simulink model "quanser_heli_IdentificadorRHONN"  (R2025a)
settings: Solver=FixedStepAuto  StartTime=0.0  StopTime=15  FixedStep=.001  RelTol=1e-3
values from neighbouring files (symbols this model uses):
  P1 = eye(2)*5e2    [ParametrosRHONN.m]
  P12 = eye(4)*5e2    [ParametrosRHONN.m]
  P2 = eye(2)*5e2    [ParametrosRHONN.m]
  P22 = eye(4)*5e2    [ParametrosRHONN.m]
  P3 = eye(2)*5e2    [ParametrosRHONN.m]
  P32 = eye(4)*5e2    [ParametrosRHONN.m]
  P4 = eye(2)*5e2    [ParametrosRHONN.m]
  P42 = eye(4)*5e2    [ParametrosRHONN.m]
  theta_0 = -40.5*pi/180    (= -0.706858347058)    [setup_heli_2d_base.m]
  VMAX_UPM_P = 24    [setup_heli_2d_base.m]
  VMAX_UPM_Y = 15    [setup_heli_2d_base.m]
  wk = zeros(8,1)    [ParametrosRHONN.m]
  wk2 = zeros(16,1)    [ParametrosRHONN.m]
undefined symbols (not defined in the file or in its folder): B_p, B_y, dspblkCoreblockFVToolHelper, g, gcbh, J_eq_p, J_eq_y, K_pp, K_py, K_yp, K_yy, l_cm, m_heli
libraries: simulink x2
settings Model: Creator=aceve  LastModifiedBy=aceve

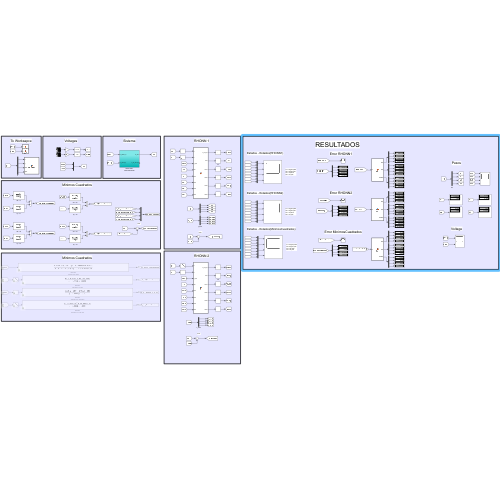
[thumbnail: Simulink's stored preview of the top-level diagram]
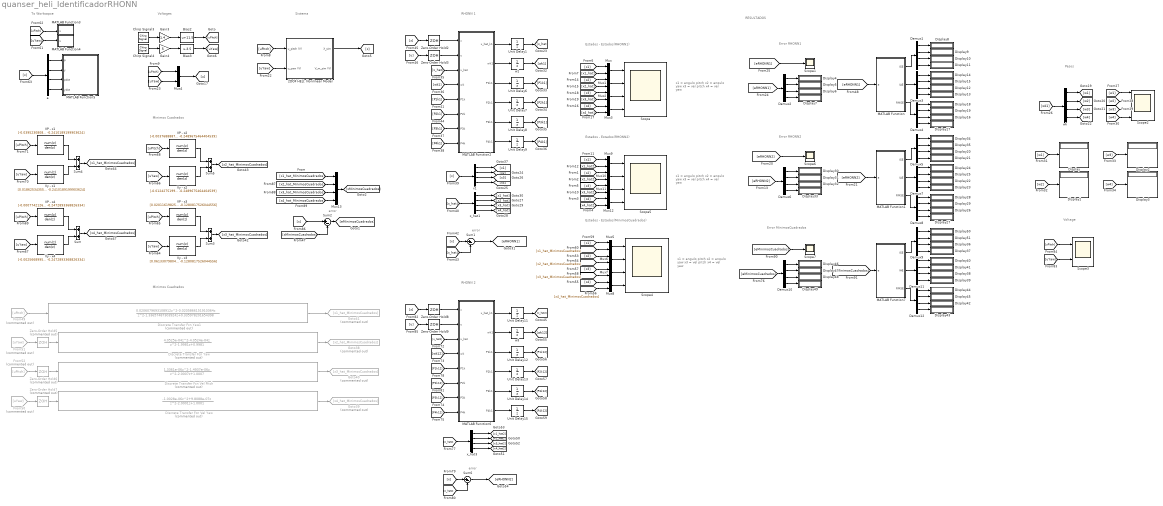
== system quanser_heli_IdentificadorRHONN ==
  note: Estados - Estados(RHONN1)
  note: Error RHONN1
  note: x1 = angulo pitch
      | x2 = angulo yaw
      | x3 = vel pitch
      | x4 = vel yaw
  note: Voltages
  note: Sistema
  note: RESULTADOS
  note: Pesos
  note: error
  note: RHONN 1
  note: Voltage
  note: Minimos Cuadrados
  note: Estados - Estados(MinimosCuadrados)
  note: x1 = angulo pitch
      | x2 = angulo yaw
      | x3 = vel pitch
      | x4 = vel yaw
  note: To Worksapce
  note: Minimos Cuadrados
  note: error
  note: RHONN 2
  note: Estados - Estados(RHONN2)
  note: x1 = angulo pitch
      | x2 = angulo yaw
      | x3 = vel pitch
      | x4 = vel yaw
  note: Error RHONN2
  note: error
  note: Error MinimosCuadrados
  2DOF HELI: Nonlinear Model : Subsystem
  Bias2 : Bias  Bias=11.5  SaturateOnIntegerOverflow=off
  Bias3 : Bias  Bias=-3.5  SaturateOnIntegerOverflow=off
  Chirp Signal3 : simulink/Sources/Chirp Signal  f1=0.08  T=10  f2=1
  Chirp Signal4 : simulink/Sources/Chirp Signal  f1=0.05  T=100  f2=1
  Demux{1..12} (12 alike) : Demux
  Discrete Transfer Fcn Vel Pitch : DiscreteTransferFcn  Commented=on  LoadFcn=dspblkCoreblockFVToolHelper(gcbh,'load');  Numerator=[1.3361e-06 -1.4937e-06 0]  Denominator=[1 -2.0007 1.0007]  a0EqualsOne=on
      settings: CopyFcn=dspblkCoreblockFVToolHelper(gcbh,'copy');  DeleteFcn=dspblkCoreblockFVToolHelper(gcbh,'close');  ModelCloseFcn=dspblkCoreblockFVToolHelper(gcbh,'close');  PreSaveFcn=dspblkCoreblockFVToolHelper(gcbh,'presave');  PostSaveFcn=dspblkCoreblockFVToolHelper(gcbh,'postsave');  CloseFcn=dspblkCoreblockFVToolHelper(gcbh,'close');
  Discrete Transfer Fcn Vel Yaw : DiscreteTransferFcn  Commented=on  LoadFcn=dspblkCoreblockFVToolHelper(gcbh,'load');  Numerator=[-1.0028e-06 9.8088e-07 0]  Denominator=[1 -2.0001 1.0001]  a0EqualsOne=on
      settings: CopyFcn=dspblkCoreblockFVToolHelper(gcbh,'copy');  DeleteFcn=dspblkCoreblockFVToolHelper(gcbh,'close');  ModelCloseFcn=dspblkCoreblockFVToolHelper(gcbh,'close');  PreSaveFcn=dspblkCoreblockFVToolHelper(gcbh,'presave');  PostSaveFcn=dspblkCoreblockFVToolHelper(gcbh,'postsave');  CloseFcn=dspblkCoreblockFVToolHelper(gcbh,'close');
  Discrete Transfer Fcn Yaw : DiscreteTransferFcn  Commented=on  LoadFcn=dspblkCoreblockFVToolHelper(gcbh,'load');  Numerator=[4.0525e-04 -4.0524e-04 0]  Denominator=[1 -1.9981 0.9981]  a0EqualsOne=on
      settings: CopyFcn=dspblkCoreblockFVToolHelper(gcbh,'copy');  DeleteFcn=dspblkCoreblockFVToolHelper(gcbh,'close');  ModelCloseFcn=dspblkCoreblockFVToolHelper(gcbh,'close');  PreSaveFcn=dspblkCoreblockFVToolHelper(gcbh,'presave');  PostSaveFcn=dspblkCoreblockFVToolHelper(gcbh,'postsave');  CloseFcn=dspblkCoreblockFVToolHelper(gcbh,'close');
  Discrete Transfer Fcn Yaw1 : DiscreteTransferFcn  Commented=on  LoadFcn=dspblkCoreblockFVToolHelper(gcbh,'load');  Numerator=[0.0206079693108912 -0.0205866151910364 0]  Denominator=[1 -1.33657487303924 0.335978201654398]  InitialStates=[-0.61509767 0.12995987]  a0EqualsOne=on
      settings: CopyFcn=dspblkCoreblockFVToolHelper(gcbh,'copy');  DeleteFcn=dspblkCoreblockFVToolHelper(gcbh,'close');  ModelCloseFcn=dspblkCoreblockFVToolHelper(gcbh,'close');  PreSaveFcn=dspblkCoreblockFVToolHelper(gcbh,'presave');  PostSaveFcn=dspblkCoreblockFVToolHelper(gcbh,'postsave');  CloseFcn=dspblkCoreblockFVToolHelper(gcbh,'close');
  Display{,1..51} (52 alike) : Display
  From49 : From  Commented=on  GotoTag=uPitch
  From50 : From  Commented=on  GotoTag=uYaw
  From51 : From  Commented=on  GotoTag=uYaw
  From52 : From  Commented=on  GotoTag=uPitch
  Gain3 : Gain  Gain=1.4
  Gain4 : Gain  Gain=5
  Goto38 : Goto  Commented=on  GotoTag=x2_hat_MinimosCuadrados
  Goto39 : Goto  Commented=on  GotoTag=x4_hat_MinimosCuadrados
  Goto40 : Goto  Commented=on  GotoTag=x3_hat_MinimosCuadrados
  Goto41 : Goto  Commented=on  GotoTag=x1_hat_MinimosCuadrados
  MATLAB Function : MATLAB Function  TreatAsAtomicUnit=on
  MATLAB Function1 : MATLAB Function  TreatAsAtomicUnit=on
  MATLAB Function2 : MATLAB Function  TreatAsAtomicUnit=on
  MATLAB Function3 : MATLAB Function  TreatAsAtomicUnit=on
  MATLAB Function4 : MATLAB Function  TreatAsAtomicUnit=on
  MATLAB Function5 : MATLAB Function  TreatAsAtomicUnit=on
  MATLAB Function6 : MATLAB Function  TreatAsAtomicUnit=on
  MATLAB Function7 : MATLAB Function  TreatAsAtomicUnit=on
  Mux{,1..12} (13 alike) : Mux  Inputs=2
  Mux13 : Mux
  Scope{,2,4..5} (4 alike) : Scope  NumInputPorts=4
      Scope settings: ActiveDisplayYMinimum=-0.84384917353702449  ActiveDisplayYMaximum=0.094948446572447137
      Scope2 settings: ActiveDisplayYMinimum=-0.70088433050936716  ActiveDisplayYMaximum=1.4334945118996132  DataLoggingVariableName=ScopeData2
      Scope4 settings: ActiveDisplayYMinimum=-0.77876884866635865  ActiveDisplayYMaximum=-0.059663832579807244  DataLoggingVariableName=ScopeData4
      Scope5 settings: ActiveDisplayYMinimum=-0.84384917353702449  ActiveDisplayYMaximum=0.094948446572447137  DataLoggingVariableName=ScopeData5
  Scope1 : Scope
      settings: ActiveDisplayYMinimum=-0.80920578422516953  ActiveDisplayYMaximum=0.12318319700603184
  Scope3 : Scope  NumInputPorts=2
      settings: ActiveDisplayYMinimum=-11.174999961452089  ActiveDisplayYMaximum=15.574999929221228  DataLoggingVariableName=ScopeData3
  Scope6 : Scope
      settings: ActiveDisplayYMinimum=-0.80920578422516953  ActiveDisplayYMaximum=0.12318319700603184  DataLoggingVariableName=ScopeData6
  Scope7 : Scope
      settings: ActiveDisplayYMinimum=-0.80920578422516953  ActiveDisplayYMaximum=0.12318319700603184  DataLoggingVariableName=ScopeData7
  Sum{,3..5} (4 alike) : Sum
  Sum1 : Sum  Inputs=|+-
  Sum2 : Sum  Inputs=|+-
  Sum6 : Sum  Inputs=|+-
  Unit Delay1 : UnitDelay  SampleTime=-1  HasFrameUpgradeWarning=on
  Unit Delay11 : UnitDelay  SampleTime=-1  HasFrameUpgradeWarning=on
  Unit Delay12 : UnitDelay  InitialCondition=P12  SampleTime=-1  HasFrameUpgradeWarning=on
  Unit Delay13 : UnitDelay  InitialCondition=P22  SampleTime=-1  HasFrameUpgradeWarning=on
  Unit Delay14 : UnitDelay  InitialCondition=P32  SampleTime=-1  HasFrameUpgradeWarning=on
  Unit Delay15 : UnitDelay  InitialCondition=P42  SampleTime=-1  HasFrameUpgradeWarning=on
  Unit Delay6 : UnitDelay  InitialCondition=P1  SampleTime=-1  HasFrameUpgradeWarning=on
  Unit Delay7 : UnitDelay  InitialCondition=P2  SampleTime=-1  HasFrameUpgradeWarning=on
  Unit Delay8 : UnitDelay  InitialCondition=P3  SampleTime=-1  HasFrameUpgradeWarning=on
  Unit Delay9 : UnitDelay  InitialCondition=P4  SampleTime=-1  HasFrameUpgradeWarning=on
  VP - x1 : DiscreteTransferFcn  LoadFcn=dspblkCoreblockFVToolHelper(gcbh,'load');  Numerator=[-0.03952308083807093 0.01457910362503944 0.0132465358893853 0.0116502395543983 0]  Denominator=[1 -0.2596941129912199 -0.2512083520588688 -0.246113610865054 -0.2410189199903624]  a0EqualsOne=on
      settings: CopyFcn=dspblkCoreblockFVToolHelper(gcbh,'copy');  DeleteFcn=dspblkCoreblockFVToolHelper(gcbh,'close');  ModelCloseFcn=dspblkCoreblockFVToolHelper(gcbh,'close');  PreSaveFcn=dspblkCoreblockFVToolHelper(gcbh,'presave');  PostSaveFcn=dspblkCoreblockFVToolHelper(gcbh,'postsave');  CloseFcn=dspblkCoreblockFVToolHelper(gcbh,'close');
  VP - x2 : DiscreteTransferFcn  LoadFcn=dspblkCoreblockFVToolHelper(gcbh,'load');  Numerator=[-0.003768888777310456 -0.001235966092478362 0.001315157335725626 0.003827291194365801 0]  Denominator=[1 -0.2509050215084465 -0.2502617960478971 -0.2496159714324903 -0.2489675464404539]  a0EqualsOne=on
      settings: CopyFcn=dspblkCoreblockFVToolHelper(gcbh,'copy');  DeleteFcn=dspblkCoreblockFVToolHelper(gcbh,'close');  ModelCloseFcn=dspblkCoreblockFVToolHelper(gcbh,'close');  PreSaveFcn=dspblkCoreblockFVToolHelper(gcbh,'presave');  PostSaveFcn=dspblkCoreblockFVToolHelper(gcbh,'postsave');  CloseFcn=dspblkCoreblockFVToolHelper(gcbh,'close');
  VP - x3 : DiscreteTransferFcn  LoadFcn=dspblkCoreblockFVToolHelper(gcbh,'load');  Numerator=[0.02011619825005108 0.006568459415468767 -0.006119667445303119 -0.02055837664883229 0]  Denominator=[1 -0.3716516698733148 -0.2906441537001457 -0.2094533609274164 -0.1280817526044556]  a0EqualsOne=on
      settings: CopyFcn=dspblkCoreblockFVToolHelper(gcbh,'copy');  DeleteFcn=dspblkCoreblockFVToolHelper(gcbh,'close');  ModelCloseFcn=dspblkCoreblockFVToolHelper(gcbh,'close');  PreSaveFcn=dspblkCoreblockFVToolHelper(gcbh,'presave');  PostSaveFcn=dspblkCoreblockFVToolHelper(gcbh,'postsave');  CloseFcn=dspblkCoreblockFVToolHelper(gcbh,'close');
  VP - x4 : DiscreteTransferFcn  LoadFcn=dspblkCoreblockFVToolHelper(gcbh,'load');  Numerator=[-0.000774212667988009 -0.0001464440180138851 0.0004853777300417859 0.001107287718628923 0]  Denominator=[1 -0.2478215083584044 -0.2476467681554213 -0.2474693715809018 -0.2472893368826334]  a0EqualsOne=on
      settings: CopyFcn=dspblkCoreblockFVToolHelper(gcbh,'copy');  DeleteFcn=dspblkCoreblockFVToolHelper(gcbh,'close');  ModelCloseFcn=dspblkCoreblockFVToolHelper(gcbh,'close');  PreSaveFcn=dspblkCoreblockFVToolHelper(gcbh,'presave');  PostSaveFcn=dspblkCoreblockFVToolHelper(gcbh,'postsave');  CloseFcn=dspblkCoreblockFVToolHelper(gcbh,'close');
  Vy - x1 : DiscreteTransferFcn  LoadFcn=dspblkCoreblockFVToolHelper(gcbh,'load');  Numerator=[0.01862534355611094 -0.002149223852187077 -0.006182902374224723 -0.01026641731777086 0]  Denominator=[1 -0.2596941129912199 -0.2512083520588688 -0.246113610865054 -0.2410189199903624]  a0EqualsOne=on
      settings: CopyFcn=dspblkCoreblockFVToolHelper(gcbh,'copy');  DeleteFcn=dspblkCoreblockFVToolHelper(gcbh,'close');  ModelCloseFcn=dspblkCoreblockFVToolHelper(gcbh,'close');  PreSaveFcn=dspblkCoreblockFVToolHelper(gcbh,'presave');  PostSaveFcn=dspblkCoreblockFVToolHelper(gcbh,'postsave');  CloseFcn=dspblkCoreblockFVToolHelper(gcbh,'close');
  Vy - x2 : DiscreteTransferFcn  LoadFcn=dspblkCoreblockFVToolHelper(gcbh,'load');  Numerator=[-0.0124275199058459 -0.004066593005302975 0.00431430457234765 0.01273262520586928 0]  Denominator=[1 -0.2509050215084465 -0.2502617960478971 -0.2496159714324903 -0.2489675464404539]  a0EqualsOne=on
      settings: CopyFcn=dspblkCoreblockFVToolHelper(gcbh,'copy');  DeleteFcn=dspblkCoreblockFVToolHelper(gcbh,'close');  ModelCloseFcn=dspblkCoreblockFVToolHelper(gcbh,'close');  PreSaveFcn=dspblkCoreblockFVToolHelper(gcbh,'presave');  PostSaveFcn=dspblkCoreblockFVToolHelper(gcbh,'postsave');  CloseFcn=dspblkCoreblockFVToolHelper(gcbh,'close');
  Vy - x3 : DiscreteTransferFcn  LoadFcn=dspblkCoreblockFVToolHelper(gcbh,'load');  Numerator=[0.06133079804282214 0.0207651122165453 -0.02048820045618499 -0.06163048150396479 0]  Denominator=[1 -0.3716516698733148 -0.2906441537001457 -0.2094533609274164 -0.1280817526044556]  a0EqualsOne=on
      settings: CopyFcn=dspblkCoreblockFVToolHelper(gcbh,'copy');  DeleteFcn=dspblkCoreblockFVToolHelper(gcbh,'close');  ModelCloseFcn=dspblkCoreblockFVToolHelper(gcbh,'close');  PreSaveFcn=dspblkCoreblockFVToolHelper(gcbh,'presave');  PostSaveFcn=dspblkCoreblockFVToolHelper(gcbh,'postsave');  CloseFcn=dspblkCoreblockFVToolHelper(gcbh,'close');
  Vy - x4 : DiscreteTransferFcn  LoadFcn=dspblkCoreblockFVToolHelper(gcbh,'load');  Numerator=[-0.002566899592150418 -0.0004840187454093538 0.001591783821110975 0.003664753148714413 0]  Denominator=[1 -0.2478215083584044 -0.2476467681554213 -0.2474693715809018 -0.2472893368826334]  a0EqualsOne=on
      settings: CopyFcn=dspblkCoreblockFVToolHelper(gcbh,'copy');  DeleteFcn=dspblkCoreblockFVToolHelper(gcbh,'close');  ModelCloseFcn=dspblkCoreblockFVToolHelper(gcbh,'close');  PreSaveFcn=dspblkCoreblockFVToolHelper(gcbh,'presave');  PostSaveFcn=dspblkCoreblockFVToolHelper(gcbh,'postsave');  CloseFcn=dspblkCoreblockFVToolHelper(gcbh,'close');
  Zero-Order Hold{2..3,8..9} (4 alike) : ZeroOrderHold  SampleTime=-1
  Zero-Order Hold5 : ZeroOrderHold  Commented=on  SampleTime=-1
  Zero-Order Hold6 : ZeroOrderHold  Commented=on  SampleTime=-1
  Zero-Order Hold7 : ZeroOrderHold  Commented=on  SampleTime=-1
  a : Demux
  w1 : UnitDelay  InitialCondition=[wk]  SampleTime=-1  HasFrameUpgradeWarning=on
  w3 : UnitDelay  InitialCondition=[wk2]  SampleTime=-1  HasFrameUpgradeWarning=on
  wk : Demux
  x1 : Demux
  x_hat1 : Demux
  x_hat3 : Demux
  wires:
  2DOF HELI: Nonlinear Model/1(X_sim) -> [x]
  Mux/1 -> Scope/1
  Mux1/1 -> Scope/2
  Mux2/1 -> Scope/3
  Mux3/1 -> Scope/4
  [x1] -> Mux/1
  [x1_hat] -> Mux/2
  [x2] -> Mux1/1
  [x2_hat] -> Mux1/2
  [x4] -> Mux3/1
  [x4_hat] -> Mux3/2
  [x3] -> Mux2/1
  [x3_hat] -> Mux2/2
  Chirp Signal3/1 -> Gain3/1
  Gain3/1 -> Bias2/1
  Chirp Signal4/1 -> Gain4/1
  Gain4/1 -> Bias3/1
  Bias2/1 -> [uPitch]
  Bias3/1 -> [uYaw]
  [uPitch] -> 2DOF HELI: Nonlinear Model/1(u_pitch (V))
  [uYaw] -> 2DOF HELI: Nonlinear Model/2(u_yaw (V))
  [uPitch] -> Mux4/1
  [uYaw] -> Mux4/2
  [eRHONN1] -> Demux2/1
  Demux2/2 -> Display5/1
  Demux2/4 -> Display7/1
  Demux2/1 -> Display4/1
  Demux2/3 -> Display6/1
  [eRHONN1] -> Scope1/1
  [wk1] -> wk/1
  wk/1 -> [w1]
  wk/2 -> [w2]
  wk/4 -> [w4]
  wk/3 -> [w3]
  [w1] -> Scope2/1
  [w2] -> Scope2/2
  [w4] -> Scope2/4
  [w3] -> Scope2/3
  [w1] -> Display/1
  [w2] -> Display1/1
  [w3] -> Display2/1
  [w4] -> Display3/1
  [x_hat] -> x_hat1/1
  MATLAB Function2/5(P3k1) -> Unit Delay8/1
  Unit Delay1/1 -> [x_hat]
  x1/2 -> [x2]
  x_hat1/3 -> [x3_hat]
  MATLAB Function2/2(wk1) -> w1/1
  [x] -> Zero-Order Hold2/1
  [x_hat] -> MATLAB Function2/3(x_hat)
  [P3k1] -> MATLAB Function2/7(P3k)
  [u] -> Zero-Order Hold3/1
  MATLAB Function2/1(x_hat_k1) -> Unit Delay1/1
  x1/4 -> [x4]
  [P2k1] -> MATLAB Function2/6(P2k)
  MATLAB Function2/6(P4k1) -> Unit Delay9/1
  x_hat1/1 -> [x1_hat]
  MATLAB Function2/4(P2k1) -> Unit Delay7/1
  Zero-Order Hold3/1 -> MATLAB Function2/2(u)
  x_hat1/4 -> [x4_hat]
  Zero-Order Hold2/1 -> MATLAB Function2/1(x)
  [x_hat] -> Sum1/2
  Unit Delay9/1 -> [P4k1]
  [wk1] -> MATLAB Function2/4(wk)
  w1/1 -> [wk1]
  [x] -> x1/1
  x1/1 -> [x1]
  x1/3 -> [x3]
  [P4k1] -> MATLAB Function2/8(P4k)
  [P1k1] -> MATLAB Function2/5(P1k)
  Sum1/1 -> [eRHONN1]
  Unit Delay7/1 -> [P2k1]
  Unit Delay8/1 -> [P3k1]
  Unit Delay6/1 -> [P1k1]
  MATLAB Function2/3(P1k1) -> Unit Delay6/1
  x_hat1/2 -> [x2_hat]
  [x] -> Sum1/1
  [uYaw] -> Scope3/2
  [uPitch] -> Scope3/1
  Mux4/1 -> [u]
  [eRHONN1] -> MATLAB Function/1(e)
  Demux1/4 -> Display11/1
  Demux1/3 -> Display10/1
  Demux1/2 -> Display9/1
  Demux1/1 -> Display8/1
  Demux3/4 -> Display13/1
  Demux3/2 -> Display15/1
  Demux3/3 -> Display12/1
  Demux3/1 -> Display14/1
  Demux4/3 -> Display16/1
  Demux4/4 -> Display17/1
  Demux4/2 -> Display19/1
  MATLAB Function/1(ISE) -> Demux1/1
  MATLAB Function/2(IAE) -> Demux3/1
  MATLAB Function/3(RMSE) -> Demux4/1
  Demux4/1 -> Display18/1
  Discrete Transfer Fcn Vel Yaw/1 -> Goto39/1
  Discrete Transfer Fcn Vel Pitch/1 -> Goto40/1
  Discrete Transfer Fcn Yaw/1 -> Goto38/1
  Mux8/1 -> Scope4/4
  [x3_hat_MinimosCuadrados] -> Mux7/2
  [x2_hat_MinimosCuadrados] -> Mux6/2
  [x3] -> Mux7/1
  Mux5/1 -> Scope4/1
  Mux7/1 -> Scope4/3
  [x2] -> Mux6/1
  [x4] -> Mux8/1
  Mux6/1 -> Scope4/2
  [x4_hat_MinimosCuadrados] -> Mux8/2
  [x1_hat_MinimosCuadrados] -> Mux5/2
  Zero-Order Hold5/1 -> Discrete Transfer Fcn Yaw/1
  Zero-Order Hold6/1 -> Discrete Transfer Fcn Vel Pitch/1
  Zero-Order Hold7/1 -> Discrete Transfer Fcn Vel Yaw/1
  [x1] -> Mux5/1
  [uPitch] -> MATLAB Function3/1(u)
  [uYaw] -> MATLAB Function4/1(u)
  [x] -> a/1
  a/1 -> MATLAB Function5/1(p)
  a/2 -> MATLAB Function5/2(y)
  a/3 -> MATLAB Function5/3(pdot)
  a/4 -> MATLAB Function5/4(ydot)
  From51/1 -> Zero-Order Hold5/1
  From50/1 -> Zero-Order Hold7/1
  From52/1 -> Zero-Order Hold6/1
  Discrete Transfer Fcn Yaw1/1 -> Goto41/1
  From49/1 -> Discrete Transfer Fcn Yaw1/1
  [uYaw] -> Vy - x4/1
  [uPitch] -> VP - x4/1
  Sum/1 -> [x4_hat_MinimosCuadrados]
  VP - x4/1 -> Sum/1
  Vy - x4/1 -> Sum/2
  [uPitch] -> VP - x3/1
  Sum3/1 -> [x3_hat_MinimosCuadrados]
  VP - x3/1 -> Sum3/1
  Vy - x3/1 -> Sum3/2
  [uYaw] -> Vy - x3/1
  [uPitch] -> VP - x1/1
  Sum4/1 -> [x1_hat_MinimosCuadrados]
  VP - x1/1 -> Sum4/1
  Vy - x1/1 -> Sum4/2
  VP - x2/1 -> Sum5/1
  [uPitch] -> VP - x2/1
  Sum5/1 -> [x2_hat_MinimosCuadrados]
  Vy - x2/1 -> Sum5/2
  [uYaw] -> Vy - x2/1
  [uYaw] -> Vy - x1/1
  w3/1 -> [wk12]
  Unit Delay13/1 -> [P2k12]
  MATLAB Function6/6(P4k1) -> Unit Delay15/1
  [x_hat2] -> Sum6/2
  Sum6/1 -> [eRHONN2]
  Unit Delay12/1 -> [P1k12]
  [u] -> Zero-Order Hold9/1
  Unit Delay11/1 -> [x_hat2]
  MATLAB Function6/4(P2k1) -> Unit Delay13/1
  x_hat3/1 -> [x1_hat2]
  Zero-Order Hold9/1 -> MATLAB Function6/2(u)
  [x] -> Sum6/1
  x_hat3/3 -> [x3_hat2]
  [x_hat2] -> x_hat3/1
  x_hat3/2 -> [x2_hat2]
  MATLAB Function6/2(wk1) -> w3/1
  [P4k12] -> MATLAB Function6/8(P4k)
  Unit Delay14/1 -> [P3k12]
  x_hat3/4 -> [x4_hat2]
  [wk12] -> MATLAB Function6/4(wk)
  [P3k12] -> MATLAB Function6/7(P3k)
  Zero-Order Hold8/1 -> MATLAB Function6/1(x)
  Unit Delay15/1 -> [P4k12]
  [P2k12] -> MATLAB Function6/6(P2k)
  [x_hat2] -> MATLAB Function6/3(x_hat)
  [P1k12] -> MATLAB Function6/5(P1k)
  MATLAB Function6/1(x_hat_k1) -> Unit Delay11/1
  MATLAB Function6/3(P1k1) -> Unit Delay12/1
  MATLAB Function6/5(P3k1) -> Unit Delay14/1
  [x] -> Zero-Order Hold8/1
  Mux11/1 -> Scope5/3
  [x2_hat2] -> Mux10/2
  Mux10/1 -> Scope5/2
  [x3] -> Mux11/1
  Mux9/1 -> Scope5/1
  [x2] -> Mux10/1
  [x4_hat2] -> Mux12/2
  [x3_hat2] -> Mux11/2
  [x4] -> Mux12/1
  [x1_hat2] -> Mux9/2
  Mux12/1 -> Scope5/4
  [x1] -> Mux9/1
  Demux5/3 -> Display20/1
  Demux6/1 -> Display30/1
  Demux5/4 -> Display21/1
  Demux7/1 -> Display24/1
  Demux5/2 -> Display35/1
  Demux8/1 -> Display28/1
  Demux8/3 -> Display26/1
  Demux6/4 -> Display33/1
  MATLAB Function1/2(IAE) -> Demux7/1
  Demux6/3 -> Display32/1
  Demux6/2 -> Display31/1
  MATLAB Function1/3(RMSE) -> Demux8/1
  Demux5/1 -> Display34/1
  Demux7/2 -> Display25/1
  [eRHONN2] -> Demux6/1
  [eRHONN2] -> MATLAB Function1/1(e)
  Demux8/4 -> Display27/1
  [eRHONN2] -> Scope6/1
  Demux7/4 -> Display23/1
  MATLAB Function1/1(ISE) -> Demux5/1
  Demux8/2 -> Display29/1
  Demux7/3 -> Display22/1
  Sum2/1 -> [eMinimosCuadrados]
  [x3_hat_MinimosCuadrados] -> Mux13/3
  [x2_hat_MinimosCuadrados] -> Mux13/2
  [x1_hat_MinimosCuadrados] -> Mux13/1
  [x4_hat_MinimosCuadrados] -> Mux13/4
  [x] -> Sum2/1
  [xMinimosCuadrados] -> Sum2/2
  [eMinimosCuadrados] -> MATLAB Function7/1(e)
  Demux11/3 -> Display38/1
  Demux12/2 -> Display45/1
  MATLAB Function7/1(ISE) -> Demux9/1
  Demux12/4 -> Display43/1
  Demux9/1 -> Display50/1
  [eMinimosCuadrados] -> Scope7/1
  [eMinimosCuadrados] -> Demux10/1
  Demux11/2 -> Display41/1
  Demux11/4 -> Display39/1
  Demux10/3 -> Display48/1
  Demux10/2 -> Display47/1
  MATLAB Function7/3(RMSE) -> Demux12/1
  Demux10/4 -> Display49/1
  Demux12/3 -> Display42/1
  Demux12/1 -> Display44/1
  Demux11/1 -> Display40/1
  Demux9/4 -> Display37/1
  Demux9/2 -> Display51/1
  Demux10/1 -> Display46/1
  MATLAB Function7/2(IAE) -> Demux11/1
  Demux9/3 -> Display36/1
  Mux13/1 -> [xMinimosCuadrados]

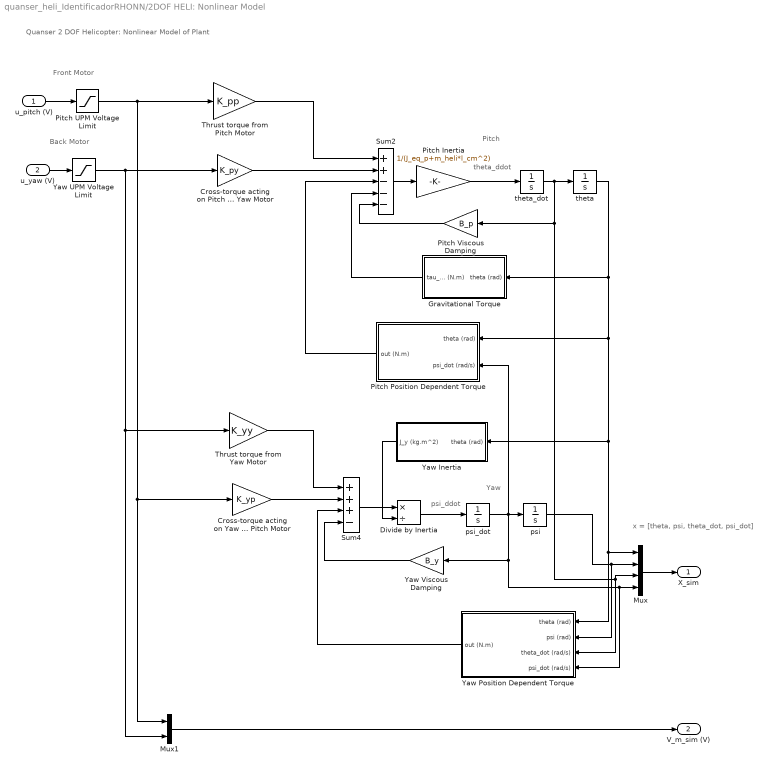
== system quanser_heli_IdentificadorRHONN/2DOF HELI: Nonlinear Model ==
  note: Back Motor
  note: Front Motor
  note: x = [theta, psi, theta_dot, psi_dot]
  note: Quanser 2 DOF Helicopter: Nonlinear Model of Plant
  note: theta_ddot
  note: psi_ddot
  note: Pitch
  note: Yaw
  u_pitch (V) : Inport
  u_yaw (V) : Inport  Port=2
  Cross-torque acting on Pitch from Yaw Motor : Gain  Gain=K_py
  Cross-torque acting on Yaw from Pitch Motor : Gain  Gain=K_yp
  Divide by Inertia : Product  Inputs=*/
  Gravitational Torque : Subsystem
  Mux : Mux
  Mux1 : Mux  Inputs=2
  Pitch Inertia : Gain  Gain=1/(J_eq_p+m_heli*l_cm^2)
  Pitch Position Dependent Torque : Subsystem  AncestorBlock=heli_2d_lib/2DOF Helicopter: Nonlinear Model/Yaw Nonlinear Element
  Pitch UPM Voltage Limit : Saturate  UpperLimit=VMAX_UPM_P  LowerLimit=- VMAX_UPM_P
  Pitch Viscous Damping : Gain  Gain=B_p
  Sum2 : Sum  Inputs=++---
  Sum4 : Sum  Inputs=+++-
  Thrust torque from Pitch Motor : Gain  Gain=K_pp
  Thrust torque from Yaw Motor : Gain  Gain=K_yy
  Yaw Inertia : Subsystem
  Yaw Position Dependent Torque : Subsystem
  Yaw UPM Voltage Limit : Saturate  UpperLimit=VMAX_UPM_Y  LowerLimit=- VMAX_UPM_Y
  Yaw Viscous Damping : Gain  Gain=B_y
  psi : Integrator
  psi_dot : Integrator
  theta : Integrator  InitialCondition=theta_0  LimitOutput=on  UpperSaturationLimit=40.5*pi/180  LowerSaturationLimit=-40.5*pi/180
  theta_dot : Integrator
  X_sim : Outport
  V_m_sim (V) : Outport  Port=2
  wires:
  Pitch Position Dependent Torque/1(out (N.m)) -> Sum2/3
  Gravitational Torque/1(tau_g (N.m)) -> Sum2/4
  Pitch Viscous Damping/1 -> Sum2/5
  Cross-torque acting on Pitch from Yaw Motor/1 -> Sum2/2
  Thrust torque from Pitch Motor/1 -> Sum2/1
  Yaw Inertia/1(J_y (kg.m^2)) -> Divide by Inertia/2
  Divide by Inertia/1 -> psi_dot/1
  Sum4/1 -> Divide by Inertia/1
  Yaw Position Dependent Torque/1(out (N.m)) -> Sum4/3
  Yaw Viscous Damping/1 -> Sum4/4
  psi/1 -> Yaw Position Dependent Torque/2(psi (rad)), Mux/2
  Mux1/1 -> V_m_sim (V)/1
  Yaw UPM Voltage Limit/1 -> Thrust torque from Yaw Motor/1, Mux1/2, Cross-torque acting on Pitch from Yaw Motor/1
  Pitch UPM Voltage Limit/1 -> Mux1/1, Cross-torque acting on Yaw from Pitch Motor/1, Thrust torque from Pitch Motor/1
  Mux/1 -> X_sim/1
  theta/1 -> Gravitational Torque/1(theta (rad)), Pitch Position Dependent Torque/1(theta (rad)), Yaw Position Dependent Torque/1(theta (rad)), Mux/1, Yaw Inertia/1(theta (rad))
  Sum2/1 -> Pitch Inertia/1
  Pitch Inertia/1 -> theta_dot/1
  theta_dot/1 -> Pitch Viscous Damping/1, Yaw Position Dependent Torque/3(theta_dot (rad/s)), Mux/3, theta/1
  Thrust torque from Yaw Motor/1 -> Sum4/1
  Cross-torque acting on Yaw from Pitch Motor/1 -> Sum4/2
  psi_dot/1 -> Yaw Viscous Damping/1, Yaw Position Dependent Torque/4(psi_dot (rad/s)), Mux/4, Pitch Position Dependent Torque/2(psi_dot (rad/s)), psi/1
  u_pitch (V)/1 -> Pitch UPM Voltage Limit/1
  u_yaw (V)/1 -> Yaw UPM Voltage Limit/1

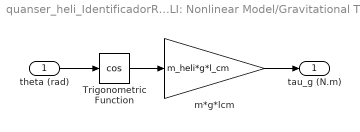
== system quanser_heli_IdentificadorRHONN/2DOF HELI: Nonlinear Model/Gravitational Torque ==
  theta (rad) : Inport
  Trigonometric Function : Trigonometry  Operator=cos  OutputSignalType=real
  m*g*lcm : Gain  Gain=m_heli*g*l_cm
  tau_g (N.m) : Outport
  wires:
  m*g*lcm/1 -> tau_g (N.m)/1
  theta (rad)/1 -> Trigonometric Function/1
  Trigonometric Function/1 -> m*g*lcm/1

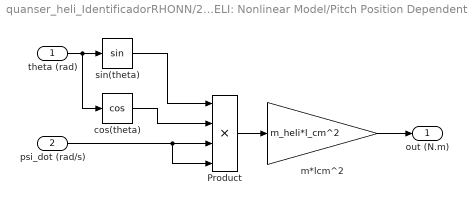
== system quanser_heli_IdentificadorRHONN/2DOF HELI: Nonlinear Model/Pitch Position Dependent Torque ==
  theta (rad) : Inport
  psi_dot (rad/s) : Inport  Port=2
  Product : Product  Inputs=4  RndMeth=Zero
  cos(theta) : Trigonometry  Operator=cos  OutputSignalType=real
  m*lcm^2 : Gain  Gain=m_heli*l_cm^2
  sin(theta) : Trigonometry  OutputSignalType=real
  out (N.m) : Outport
  wires:
  psi_dot (rad/s)/1 -> Product/4, Product/3
  theta (rad)/1 -> cos(theta)/1, sin(theta)/1
  Product/1 -> m*lcm^2/1
  sin(theta)/1 -> Product/1
  cos(theta)/1 -> Product/2
  m*lcm^2/1 -> out (N.m)/1

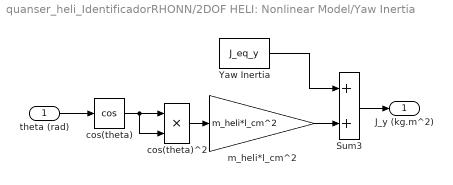
== system quanser_heli_IdentificadorRHONN/2DOF HELI: Nonlinear Model/Yaw Inertia ==
  theta (rad) : Inport
  Sum3 : Sum
  Yaw Inertia : Constant  Value=J_eq_y
  cos(theta) : Trigonometry  Operator=cos  OutputSignalType=real
  cos(theta)^2 : Product  RndMeth=Zero
  m_heli*l_cm^2 : Gain  Gain=m_heli*l_cm^2
  J_y (kg.m^2) : Outport
  wires:
  cos(theta)/1 -> cos(theta)^2/2, cos(theta)^2/1
  Sum3/1 -> J_y (kg.m^2)/1
  theta (rad)/1 -> cos(theta)/1
  m_heli*l_cm^2/1 -> Sum3/2
  Yaw Inertia/1 -> Sum3/1
  cos(theta)^2/1 -> m_heli*l_cm^2/1

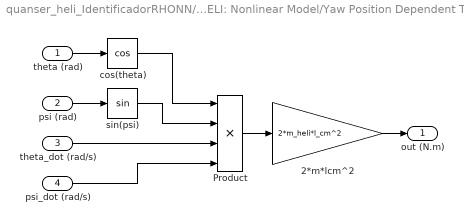
== system quanser_heli_IdentificadorRHONN/2DOF HELI: Nonlinear Model/Yaw Position Dependent Torque ==
  theta (rad) : Inport
  psi (rad) : Inport  Port=2
  theta_dot (rad/s) : Inport  Port=3
  psi_dot (rad/s) : Inport  Port=4
  2*m*lcm^2 : Gain  Gain=2*m_heli*l_cm^2
  Product : Product  Inputs=4  RndMeth=Zero
  cos(theta) : Trigonometry  Operator=cos  OutputSignalType=real
  sin(psi) : Trigonometry  OutputSignalType=real
  out (N.m) : Outport
  wires:
  2*m*lcm^2/1 -> out (N.m)/1
  psi_dot (rad/s)/1 -> Product/4
  theta_dot (rad/s)/1 -> Product/3
  sin(psi)/1 -> Product/2
  cos(theta)/1 -> Product/1
  Product/1 -> 2*m*lcm^2/1
  theta (rad)/1 -> cos(theta)/1
  psi (rad)/1 -> sin(psi)/1

== matlab function quanser_heli_IdentificadorRHONN/MATLAB Function1 ==
  settings: updateMethod=DISCRETE
  data: e input; ISE output; IAE output; RMSE output
function [ISE, IAE, RMSE] = fcn(e)
% Entrada:
%   e   : vector 4x1 con errores [e1;e2;e3;e4]
% Salidas (todas 4x1 para Demux de 4):
%   ISE : integral del error cuadrático por estado
%   IAE : integral del error absoluto por estado
%   RMSE: raíz del error cuadrático medio por estado

% --- fija tamaños para Simulink ---
ISE  = zeros(4,1);
IAE  = zeros(4,1);
RMSE = zeros(4,1);

% --- periodo de muestreo (ajústalo) ---
Ts = 0.001;

% --- fuerza forma 4x1 ---
e = reshape(e,4,1);

% --- acumuladores persistentes por estado ---
persistent S_ISE S_IAE S_E2 N
if isempty(S_ISE)
    S_ISE = zeros(4,1);
    S_IAE = zeros(4,1);
    S_E2  = zeros(4,1);
    N     = uint32(0);
end

% --- actualizar métricas ---
S_ISE = S_ISE + (e.^2)*Ts;   % ISE_i = ∫ e_i^2 dt
S_IAE = S_IAE + abs(e)*Ts;   % IAE_i = ∫ |e_i| dt
S_E2  = S_E2  + (e.^2);      % para RMSE_i
N     = N + 1;

% --- salidas ---
ISE  = S_ISE;
IAE  = S_IAE;
RMSE = sqrt( S_E2 ./ max(1,double(N)) );  % promedio por muestra

end

== matlab function quanser_heli_IdentificadorRHONN/MATLAB Function2 ==
  data: x input; u input; x_hat_k1 output; x_hat input; wk input; P1k input; P2k input; wk1 output; P1k1 output; P2k1 output; P3k input; P4k input; P3k1 output; P4k1 output
function [x_hat_k1, wk1, P1k1, P2k1, P3k1, P4k1] = fcn(x,u,x_hat,wk,P1k,P2k,P3k,P4k)
% Identificador RHONN con 4 EKF (uno por estado)
% x = [x1; x2; x3; x4], u = [u1; u2]
% wk = [w1 w2 | w3 w4 | w5 w6 | w7 w8]'

%% Ganancias constantes de entrada (ajustables)
O1 = 0.01;
O2 = 0.01;

%% Modelo neuronal (predicción x_hat(k+1))
x_hat_1 = wk(1)*tanh(x(3)) + wk(2)*tanh(x(1));
x_hat_2 = wk(3)*tanh(x(4)) + wk(4)*tanh(x(2));
x_hat_3 = wk(5)*tanh(x(3)) + wk(6)*tanh(x(1)) + O1*u(1);
x_hat_4 = wk(7)*tanh(x(4)) + wk(8)*tanh(x(2)) + O2*u(2);
x_hat_k1 = [x_hat_1; x_hat_2; x_hat_3; x_hat_4];

%% Regresores (derivadas parciales respecto a wk)
H1 = [tanh(x(3)) tanh(x(1))];
H2 = [tanh(x(4)) tanh(x(2))];
H3 = [tanh(x(3)) tanh(x(1))];
H4 = [tanh(x(4)) tanh(x(2))];

%% Covarianzas EKF
Q1 = eye(2)*5e2;  R1 = 6e3;
Q2 = eye(2)*1e2;  R2 = 6e1;
Q3 = eye(2)*5e2;  R3 = 6e3;
Q4 = eye(2)*5e2;  R4 = 6e2;

%% Innovación
e = x - x_hat;

%% EKF #1 (actualiza [w1 w2])
K1   = P1k*H1'/(R1 + H1*P1k*H1');
w1k1 = [wk(1); wk(2)] + K1*e(1);
P1k1 = P1k - K1*H1*P1k + Q1;

%% EKF #2 (actualiza [w3 w4])
K2   = P2k*H2'/(R2 + H2*P2k*H2');
w2k1 = [wk(3); wk(4)] + K2*e(2);
P2k1 = P2k - K2*H2*P2k + Q2;

%% EKF #3 (actualiza [w5 w6])
K3   = P3k*H3'/(R3 + H3*P3k*H3');
w3k1 = [wk(5); wk(6)] + K3*e(3);
P3k1 = P3k - K3*H3*P3k + Q3;

%% EKF #4 (actualiza [w7 w8])
K4   = P4k*H4'/(R4 + H4*P4k*H4');
w4k1 = [wk(7); wk(8)] + K4*e(4);
P4k1 = P4k - K4*H4*P4k + Q4;

%% Ensamble de pesos
wk1 = [w1k1; w2k1; w3k1; w4k1];



end

== matlab function quanser_heli_IdentificadorRHONN/MATLAB Function ==
  settings: updateMethod=DISCRETE
  data: e input; ISE output; IAE output; RMSE output
function [ISE, IAE, RMSE] = fcn(e)
% Entrada:
%   e   : vector 4x1 con errores [e1;e2;e3;e4]
% Salidas (todas 4x1 para Demux de 4):
%   ISE : integral del error cuadrático por estado
%   IAE : integral del error absoluto por estado
%   RMSE: raíz del error cuadrático medio por estado

% --- fija tamaños para Simulink ---
ISE  = zeros(4,1);
IAE  = zeros(4,1);
RMSE = zeros(4,1);

% --- periodo de muestreo (ajústalo) ---
Ts = 0.001;

% --- fuerza forma 4x1 ---
e = reshape(e,4,1);

% --- acumuladores persistentes por estado ---
persistent S_ISE S_IAE S_E2 N
if isempty(S_ISE)
    S_ISE = zeros(4,1);
    S_IAE = zeros(4,1);
    S_E2  = zeros(4,1);
    N     = uint32(0);
end

% --- actualizar métricas ---
S_ISE = S_ISE + (e.^2)*Ts;   % ISE_i = ∫ e_i^2 dt
S_IAE = S_IAE + abs(e)*Ts;   % IAE_i = ∫ |e_i| dt
S_E2  = S_E2  + (e.^2);      % para RMSE_i
N     = N + 1;

% --- salidas ---
ISE  = S_ISE;
IAE  = S_IAE;
RMSE = sqrt( S_E2 ./ max(1,double(N)) );  % promedio por muestra

end

== matlab function quanser_heli_IdentificadorRHONN/MATLAB Function3 ==
  settings: updateMethod=DISCRETE
  data: u input
function log_Vp(u)
%#codegen
% Discreto a Ts=0.001 s. Escribe Vp_log=[t u] en base.
coder.extrinsic('assignin');
Ts = coder.const(0.001);

persistent k T Y
if isempty(k); k = uint32(0); T = zeros(0,1); Y = zeros(0,1); end

k = k + 1;                 % contador de muestras
t = double(k-1) * Ts;      % tiempo discreto

T = [T; t];
Y = [Y; u];

assignin('base','Vp_log',[T Y]);
end

== matlab function quanser_heli_IdentificadorRHONN/MATLAB Function4 ==
  settings: updateMethod=DISCRETE
  data: u input
function log_Vy(u)
%#codegen
% Discreto a Ts=0.001 s. Escribe Vy_log=[t u] en base.
coder.extrinsic('assignin');
Ts = coder.const(0.001);

persistent k T Y
if isempty(k); k = uint32(0); T = zeros(0,1); Y = zeros(0,1); end

k = k + 1;
t = double(k-1) * Ts;

T = [T; t];
Y = [Y; u];

assignin('base','Vy_log',[T Y]);
end

== matlab function quanser_heli_IdentificadorRHONN/MATLAB Function5 ==
  settings: updateMethod=DISCRETE
  data: p input; y input; pdot input; ydot input
function log_states(p, y, pdot, ydot)
%#codegen
% Discreto a Ts=0.001 s. Escribe:
%  p_log=[t p], pdot_log=[t pdot], y_log=[t y], ydot_log=[t ydot]
coder.extrinsic('assignin');
Ts = coder.const(0.001);

persistent k T P PD Y YD
if isempty(k)
    k  = uint32(0);
    T  = zeros(0,1);  P  = zeros(0,1);
    PD = zeros(0,1);  Y  = zeros(0,1);  YD = zeros(0,1);
end

k = k + 1;
t = double(k-1) * Ts;

T  = [T;  t];
P  = [P;  p];
PD = [PD; pdot];
Y  = [Y;  y];
YD = [YD; ydot];

assignin('base','p_log',    [T P ]);
assignin('base','pdot_log', [T PD]);
assignin('base','y_log',    [T Y ]);
assignin('base','ydot_log', [T YD]);
end

== matlab function quanser_heli_IdentificadorRHONN/MATLAB Function6 ==
  data: x input; u input; x_hat_k1 output; x_hat input; wk input; P1k input; P2k input; wk1 output; P1k1 output; P2k1 output; P3k input; P4k input; P3k1 output; P4k1 output
function [x_hat_k1, wk1, P1k1, P2k1, P3k1, P4k1] = fcn(x,u,x_hat,wk,P1k,P2k,P3k,P4k)
% RHONN + 4 EKF (uno por estado) con 4 pesos/estado = 16 pesos total
% x=[x1;x2;x3;x4], u=[u1;u2], wk=[w1..w4|w5..w8|w9..w12|w13..w16]'

% === Ganancias de entrada (fijas) ===
O1 = 0.01; O2 = 0.01;

% (opcional) anti-saturación suave para las bases
xc = max(min(x,5),-5);



% === Bases (regresores) 1×4 por estado ===
H1 = [tanh(xc(3)), tanh(xc(1)), ((xc(3)-xc(1))./(1+abs(xc(3)-xc(1)))), exp(-0.5*(xc(2)/1.0)^2)];
H2 = [tanh(xc(4)), tanh(xc(2)), ((xc(4)-xc(2))./(1+abs(xc(4)-xc(2)))), exp(-0.5*(xc(1)/1.0)^2)];
H3 = [tanh(xc(3)), tanh(xc(1)), log1p(exp(xc(3)-xc(1))),              exp(-0.5*(xc(4)/1.0)^2)];
H4 = [tanh(xc(4)), tanh(xc(2)), log1p(exp(xc(4)-xc(2))),              exp(-0.5*(xc(3)/1.0)^2)];

% === Partición de pesos (4 por estado) ===
w1 = wk(1:4);   w2 = wk(5:8);   w3 = wk(9:12);   w4 = wk(13:16);

% === Predicción x_hat(k+1) con pesos "a priori" ===
x_hat_1 = w1(1)*tanh(xc(3)) + w1(2)*tanh(0.9*xc(1)) + w1(3)*((xc(3)-xc(1))./(1+abs(xc(3)-xc(1)))) + w1(4)*exp(-0.5*(xc(2)/1.0)^2);
x_hat_2 = w2(1)*tanh(xc(4)) + w2(2)*tanh(0.9*xc(2)) + w2(3)*((xc(4)-xc(2))./(1+abs(xc(4)-xc(2)))) + w2(4)*exp(-0.5*(xc(1)/1.0)^2);
x_hat_3 = w3(1)*tanh(0.8*xc(3)) + w3(2)*tanh(0.6*xc(1)) + w3(3)*log1p(exp(xc(3)-xc(1))) + w3(4)*exp(-0.5*(xc(4)/1.0)^2) + O1*u(1);
x_hat_4 = w4(1)*tanh(0.8*xc(4)) + w4(2)*tanh(0.6*xc(2)) + w4(3)*log1p(exp(xc(4)-xc(2))) + w4(4)*exp(-0.5*(xc(3)/1.0)^2) + O2*u(2);
x_hat_k1 = [x_hat_1; x_hat_2; x_hat_3; x_hat_4];

% === Innovación ===
e = x - x_hat;   % 4x1

% === Ruido proceso/medición (ajustables) ===
Q1 = eye(4)*1e2;  R1 = 1e3;
Q2 = eye(4)*1e2;  R2 = 1e3;
Q3 = eye(4)*1e2;  R3 = 1e3;
Q4 = eye(4)*1e2;  R4 = 1e3;

% === EKF por estado (H:1x4, P:4x4, K:4x1) ===
% #1
S1  = R1 + H1*P1k*H1.';
K1  = (P1k*H1.')/S1;
w1k1 = w1 + K1*e(1);
P1k1 = P1k - K1*(H1*P1k) + Q1;     % forma simple (puedes usar Joseph si quieres)

% #2
S2  = R2 + H2*P2k*H2.';
K2  = (P2k*H2.')/S2;
w2k1 = w2 + K2*e(2);
P2k1 = P2k - K2*(H2*P2k) + Q2;

% #3
S3  = R3 + H3*P3k*H3.';
K3  = (P3k*H3.')/S3;
w3k1 = w3 + K3*e(3);
P3k1 = P3k - K3*(H3*P3k) + Q3;

% #4
S4  = R4 + H4*P4k*H4.';
K4  = (P4k*H4.')/S4;
w4k1 = w4 + K4*e(4);
P4k1 = P4k - K4*(H4*P4k) + Q4;

% === Ensamble de pesos actualizados ===
wk1 = [w1k1; w2k1; w3k1; w4k1];
end

== matlab function quanser_heli_IdentificadorRHONN/MATLAB Function7 ==
  settings: updateMethod=DISCRETE
  data: e input; ISE output; IAE output; RMSE output
function [ISE, IAE, RMSE] = fcn(e)
% Entrada:
%   e   : vector 4x1 con errores [e1;e2;e3;e4]
% Salidas (todas 4x1 para Demux de 4):
%   ISE : integral del error cuadrático por estado
%   IAE : integral del error absoluto por estado
%   RMSE: raíz del error cuadrático medio por estado

% --- fija tamaños para Simulink ---
ISE  = zeros(4,1);
IAE  = zeros(4,1);
RMSE = zeros(4,1);

% --- periodo de muestreo (ajústalo) ---
Ts = 0.001;

% --- fuerza forma 4x1 ---
e = reshape(e,4,1);

% --- acumuladores persistentes por estado ---
persistent S_ISE S_IAE S_E2 N
if isempty(S_ISE)
    S_ISE = zeros(4,1);
    S_IAE = zeros(4,1);
    S_E2  = zeros(4,1);
    N     = uint32(0);
end

% --- actualizar métricas ---
S_ISE = S_ISE + (e.^2)*Ts;   % ISE_i = ∫ e_i^2 dt
S_IAE = S_IAE + abs(e)*Ts;   % IAE_i = ∫ |e_i| dt
S_E2  = S_E2  + (e.^2);      % para RMSE_i
N     = N + 1;

% --- salidas ---
ISE  = S_ISE;
IAE  = S_IAE;
RMSE = sqrt( S_E2 ./ max(1,double(N)) );  % promedio por muestra

end
